simulink model "Task_4"  (R2016a)
settings: Solver=VariableStepAuto  StartTime=0.0  StopTime=100.0  RelTol=1e-3
undefined symbols (not defined in the file or in its folder): kd, ki, kp
libraries: simulink x1
settings Model: DataDictionary=data.sldd  Creator=Admin  LastModifiedBy=Admin

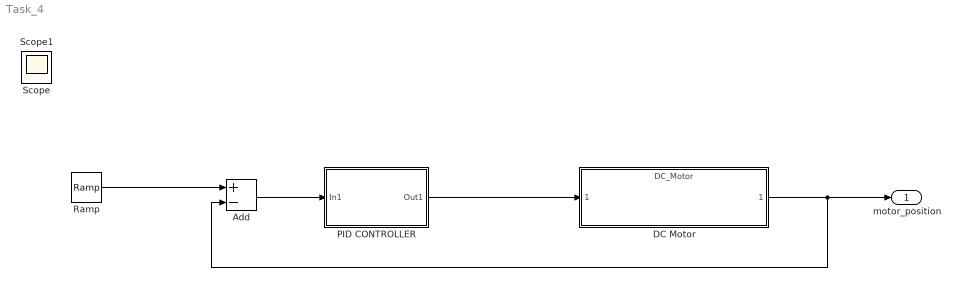
== system Task_4 ==
  Add : Sum  Inputs=+-
  "DC Motor " : ModelReference  ModelNameDialog=DC_Motor  SimulationMode=Normal  ModelReferenceVersion=1.6
  PID CONTROLLER : Subsystem
  Ramp : simulink/Sources/Ramp  slope=1  start=0  X0=0
  motor_position : Outport
  Scope : Scope
  Scope1 : Scope
  wires:
  "DC Motor "/1 -> Add/2, motor_position/1
  Ramp/1 -> Add/1
  Add/1 -> PID CONTROLLER/1(In1)
  PID CONTROLLER/1(Out1) -> "DC Motor "/1

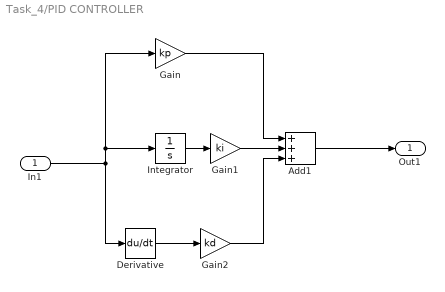
== system Task_4/PID CONTROLLER ==
  In1 : Inport
  Add1 : Sum  Inputs=+++
  Derivative : Derivative
  Gain : Gain  Gain=kp
  Gain1 : Gain  Gain=ki
  Gain2 : Gain  Gain=kd
  Integrator : Integrator
  Out1 : Outport
  wires:
  Gain2/1 -> Add1/3
  In1/1 -> Derivative/1, Integrator/1, Gain/1
  Add1/1 -> Out1/1
  Derivative/1 -> Gain2/1
  Integrator/1 -> Gain1/1
  Gain1/1 -> Add1/2
  Gain/1 -> Add1/1
